simulink model "1A"  (R2018a)
settings: Solver=VariableStepAuto  StartTime=0.0  StopTime=10.0  RelTol=1e-3
settings Model: Creator=Kamil  LastModifiedBy=Kamil

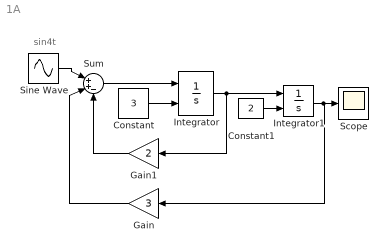
== system 1A ==
  note: sin4t
  Constant : Constant  Value=3
  Constant1 : Constant  Value=2
  Gain : Gain  Gain=3
  Gain1 : Gain  Gain=2
  Integrator : Integrator  InitialConditionSource=external  InitialCondition=3
  Integrator1 : Integrator  InitialConditionSource=external  InitialCondition=2
  Scope : Scope
  Sine Wave : Sin  Frequency=2  SampleTime=0
  Sum : Sum  Inputs=|++-
  wires:
  Sine Wave/1 -> Sum/1
  Integrator/1 -> Integrator1/1, Gain1/1
  Integrator1/1 -> Gain/1, Scope/1
  Gain/1 -> Sum/2
  Gain1/1 -> Sum/3
  Constant1/1 -> Integrator1/2
  Constant/1 -> Integrator/2
  Sum/1 -> Integrator/1
